simulink model "ciccio_ciccio (1)"  (R2022b)
settings: Solver=VariableStepAuto  StartTime=0.0  StopTime=40  FixedStep=0.01  RelTol=1e-3
values from neighbouring files (symbols this model uses):
  C1 = 5    [Modello_idraulico.m]    (also in ciccio_ciccio.m = 0.1; tesina.m = 50)
  C2 = 10    [Modello_idraulico.m]    (also in ciccio_ciccio.m = 1; tesina.m = 25)
  R1 = 0.1    [ciccio_ciccio.m]    (also in modello_termico.m = 1)
  R2 = 10    [ciccio_ciccio.m]    (also in modello_termico.m)
settings Model: Creator=frvas  LastModifiedBy=frvas

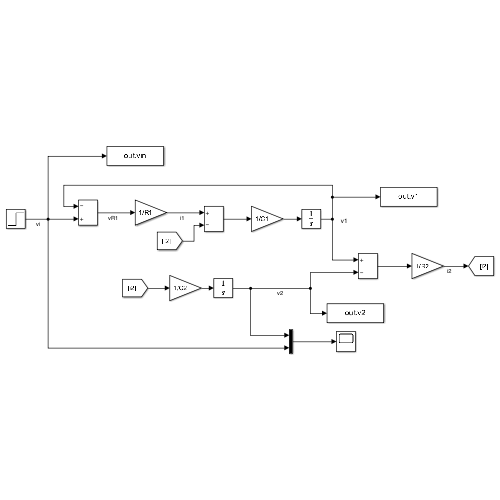
[thumbnail: Simulink's stored preview of the top-level diagram]
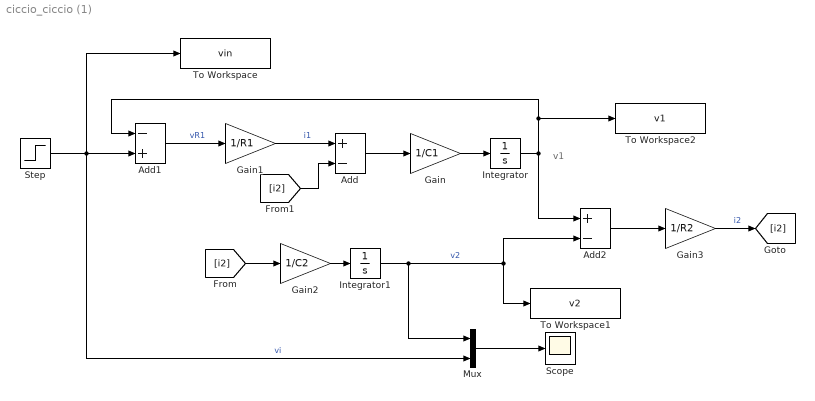
== system ciccio_ciccio (1) ==
  note: v1
  Add : Sum  Inputs=+-
  Add1 : Sum  Inputs=-+
  Add2 : Sum  Inputs=+-
  Gain : Gain  Gain=1/C1
  Gain1 : Gain  Gain=1/R1
  Gain2 : Gain  Gain=1/C2
  Gain3 : Gain  Gain=1/R2
  Integrator : Integrator
  Integrator1 : Integrator
  Mux : Mux  Inputs=2
  Scope : Scope
  Step : Step  After=7  SampleTime=0
  To Workspace : ToWorkspace  VariableName=vin  SaveFormat=Structure With Time  SampleTime=-1
  To Workspace1 : ToWorkspace  VariableName=v2  SaveFormat=Structure With Time  SampleTime=-1
  To Workspace2 : ToWorkspace  VariableName=v1  SaveFormat=Structure With Time  SampleTime=-1
  wires:
  Integrator/1 -> Add2/1, To Workspace2/1, Add1/1
  Gain/1 -> Integrator/1
  Add/1 -> Gain/1
  Gain1/1 -> Add/1  "i1"
  Add1/1 -> Gain1/1  "vR1"
  Step/1 -> To Workspace/1, Mux/2, Add1/2  "vi"
  Integrator1/1 -> Mux/1, To Workspace1/1, Add2/2  "v2"
  Gain2/1 -> Integrator1/1
  Add2/1 -> Gain3/1
  Mux/1 -> Scope/1
  Gain3/1 -> [i2]  "i2"
  [i2] -> Gain2/1
  [i2] -> Add/2
